simulink model "testBusArray"  (R2014a)
settings: Solver=FixedStepDiscrete  StartTime=0.0  StopTime=Inf  FixedStep=0.001  RelTol=1e-3
undefined symbols (not defined in the file or in its folder): serializedBusArray
libraries: dspswit3 x2, libButtons x1, simulink x1
settings Model: BufferReuse=off  Creator=Dan  LastModifiedBy=djoshea
settings SolverCC: EnableConcurrentExecution=on
settings OptimizationCC: BlockReduction=off  OptimizeBlockIOStorage=off  BufferReuse=off  GlobalBufferReuse=off  ExpressionFolding=off  LocalBlockOutputs=off
settings HardwareCC: ProdIntDivRoundTo=Zero  ProdEndianess=LittleEndian  ProdHWDeviceType=Generic->32-bit x86 compatible
settings RTWCC: SystemTargetFile=slrt.tlc  TemplateMakefile=slrt_default_tmf  Description=Simulink Real-Time  ProcessScript=slrt_make_rtw_hook  RTWCompilerOptimization=On
settings TargetCC: CodeReplacementLibrary=XPC_BLAS  ParMdlRefBuildCompliant=on  ConcurrentExecutionCompliant=on  MatFileLogging=on  EnableShiftOperators=on  MATLABClassNameForMDSCustomization=xpcAperiodicCustomization

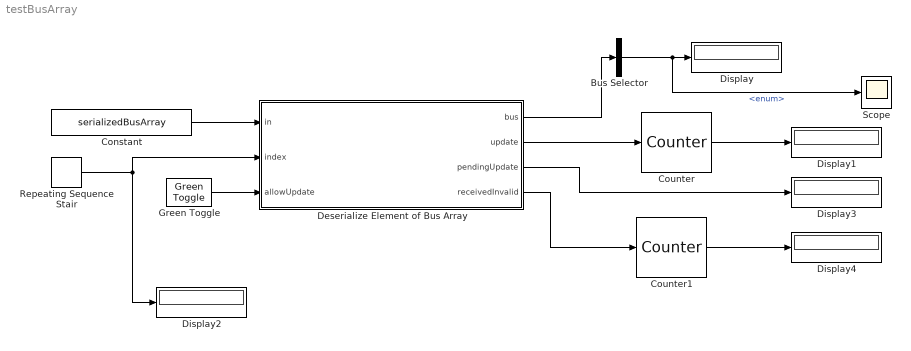
== system testBusArray ==
  Bus Selector : BusSelector  OutputSignals=enum
  Constant : Constant  Value=serializedBusArray  OutDataTypeStr=uint8
  Counter : dspswit3/Counter  Direction=Up  CountEvent=Non-zero sample  CounterSize=32 bits  MaxCount=255  InitialCount=0  Output=Count  HitValue=32  ResetInput=off  SamplesPerFrame=1  Ts=1  CntDtype=uint32  HitDtype=Logical
  Counter1 : dspswit3/Counter  Direction=Up  CountEvent=Non-zero sample  CounterSize=32 bits  MaxCount=255  InitialCount=0  Output=Count  HitValue=32  ResetInput=off  SamplesPerFrame=1  Ts=1  CntDtype=uint32  HitDtype=Logical
  Deserialize Element of Bus Array : MATLAB Function  TreatAsAtomicUnit=on  mask(BusSerialize: deserialize a single element of a serialized bus array){busType=Bus: TestBus}
      mask prompts: busType "Bus Type:"
      mask help:
      | Given a bus array serialized with BusSerialize.serializeVariableLengthBusArray, this block deserializes a specific element of that bus array. This allows bus arrays to be deserialized even when the bus contains variable length elements (or the array is of variable length), which implies that Simulink cannot currently handle the bus array.
      |
      | Select the bus type below to deserialize into.
      mask init:
      | BusSerialize.maskDeserializeVariableLengthBusArrayBlockUpdate(gcb)
  Display{,1..4} (5 alike) : Display
  Green Toggle : libButtons/Green Toggle  SystemSampleTime=-1
  Repeating Sequence Stair : simulink/Sources/Repeating Sequence Stair  OutValues=[1 2 3]'  tsamp=0.001  OutMin=[]  OutMax=[]  OutDataTypeStr=uint16  OutputDataTypeScalingMode=uint16  OutDataType=fixdt(0,8)  ConRadixGroup=Best Precision: Vector-wise  OutScaling=2^-12
  Scope : Scope
      settings: TimeRange=100
  wires:
  Constant/1 -> Deserialize Element of Bus Array/1(in)
  Repeating Sequence Stair/1 -> Display2/1, Deserialize Element of Bus Array/2(index)
  Deserialize Element of Bus Array/1(bus) -> Bus Selector/1
  Bus Selector/1 -> Scope/1, Display/1  "<enum>"
  Deserialize Element of Bus Array/2(update) -> Counter/1
  Green Toggle/1 -> Deserialize Element of Bus Array/3(allowUpdate)
  Deserialize Element of Bus Array/3(pendingUpdate) -> Display3/1
  Deserialize Element of Bus Array/4(receivedInvalid) -> Counter1/1
  Counter1/1 -> Display4/1
  Counter/1 -> Display1/1

== matlab function testBusArray/Deserialize Element of Bus Array ==
  data: in input uint8; bus output Bus: TestBus size=1; index input uint16 size=1; update output uint8 size=1; allowUpdate input uint8 size=1; pendingUpdate output uint8 size=1; receivedInvalid output uint8 size=1
function [bus, update, pendingUpdate, receivedInvalid] = deserializeBusArrayElement(in, index, allowUpdate)
%#codegen

    update = uint8(0);
    receivedInvalid = uint8(0);
    valid = uint8(0);
    changed = uint8(0);

    % only deserialize when inputs change
    persistent pIn;
    persistent pIndex;
    persistent pBus;
    persistent pPendingUpdate;
    
    % cache inputs for change detection
    if isempty(pIn)
        pIn = in;
        changed = uint8(1);
    end
    if isempty(pIndex)
        pIndex = index;
        changed = uint8(1);
    end
    
    % cache outputs so that we only update when allowUpdate is high
    if isempty(pBus)
        pBus = testBusArrayLib.initializeBus_TestBus();        
        changed = uint8(1);
    end
    if isempty(pPendingUpdate)
        pPendingUpdate = uint8(0);
    end
    
    % inputs changed?
    if ~isequal(in, pIn) || ~isequal(index, pIndex)
        changed = uint8(1);
    end
    
    % update cached inputs on change
    if changed
        pIn = in;
        pIndex = index;
        pPendingUpdate = uint8(1);
    end
    
    % deserialize a new output if we're allowing updates
    if pPendingUpdate && allowUpdate
        % length is first uint16
        N = typecast(in(1:2), 'uint16');
        if index <= N
            % followed by N uint16s indicating where each element starts
            idxOffset = uint16(index)*uint16(2) + uint16(1);
            if idxOffset <= length(in) % too short to hold that many?

                % get the offset where the requested bus element starts
                offset = typecast(in(idxOffset : (idxOffset + 1)), 'uint16');
                if offset <= length(in) % offset invalid?

                    % and deserialize the bus from that offset
                    [bus, valid] = testBusArrayLib.deserializeBus_TestBus(in, offset);
                    if valid
                        pBus = bus;
                        update = uint8(1);
                    end
                end
            end
        end

        pPendingUpdate = uint8(0);
        if ~valid
            receivedInvalid = uint8(1);
        end
    end

    bus = pBus;
    pendingUpdate = pPendingUpdate;
end
